simulink model "sampleModel2088"  (R2023a)
settings: Solver=VariableStepAuto  StartTime=0.0  StopTime=10.0  RelTol=1e-3
libraries: simulink x4, hdlsllib x4
settings Model: Creator=user1  LastModifiedBy=user1

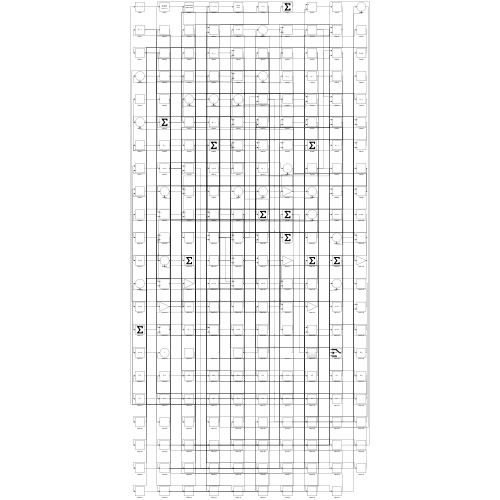
[thumbnail: Simulink's stored preview of the top-level diagram]
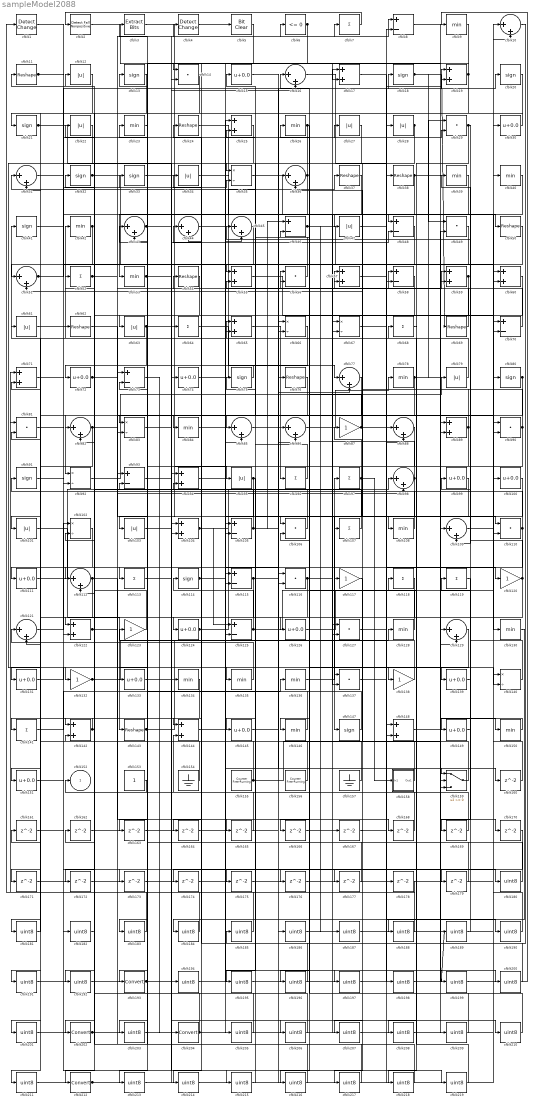
== system sampleModel2088 ==
  cfblk1 : simulink/Logic and Bit Operations/Detect Change  vinit=0  OutDataTypeStr=boolean
      settings: LibrarySourceBlock=|
      | hdlsllib/Logic and Bit
      | Operations/Detect
      | Change
  cfblk{10,16,31,36,43..45,51,77,82,85..86,88,98,109,112,121,129} (18 alike) : Sum  Inputs=|++
  cfblk{15,30,72,74,99..100,111,124,126,131,133,139,145,149,151} (15 alike) : Bias  Bias=0.0  SaturateOnIntegerOverflow=off
  cfblk{12,22,27..28,34,47,61,63,79,95,101,103} (12 alike) : Abs  SaturateOnIntegerOverflow=off
  cfblk{35,66..67,83,92,102,140} (7 alike) : Product  Inputs=*/  RndMeth=Zero  SaturateOnIntegerOverflow=on
  cfblk{17,19,25,55,57,59..60,65,71,89,94,104,122,142,144,148} (16 alike) : Sum
  cfblk{8,46,48,58,70,73,93,105,115,125} (10 alike) : Sum  Inputs=+-
  cfblk{14,29,49,56,81,90,106,110,116,127,137} (11 alike) : DotProduct  OutDataTypeStr=Inherit: Inherit via internal rule
  cfblk{7,52,64,68,96..97,107,113,118..119,141} (11 alike) : Sum  Inputs=+
  cfblk{9,23,26,39..40,42,53,78,84,108,128,130,134..136,146,150} (17 alike) : MinMax
  cfblk{11,24,37..38,50,54,62,69,76,143} (10 alike) : Reshape
  cfblk{13,18,20..21,32..33,41,75,80,91,114,147} (12 alike) : Signum
  cfblk{87,117,120,123,132,138} (6 alike) : Gain
  cfblk153 : Constant  SampleTime=-1
  cfblk154 : Ground
  cfblk155 : hdlsllib/Sources/Counter Free-Running  NumBits=16  tsamp=-1
  cfblk156 : hdlsllib/Sources/Counter Free-Running  NumBits=16  tsamp=-1
  cfblk157 : Ground
  cfblk158 : Subsystem
      settings: LibrarySourceBlock=|
      | hdlsllib/Ports &
      | Subsystems/Subsystem
  cfblk159 : Switch  SaturateOnIntegerOverflow=off  InputSameDT=off
  cfblk{160..179} (20 alike) : Delay  SampleTime=1
  cfblk{180..192,194..201,203,205..211,213..219} (36 alike) : DataTypeConversion  OutDataTypeStr=uint8  SaturateOnIntegerOverflow=off  RndMeth=Floor
  cfblk{193,202,204,212} (4 alike) : DataTypeConversion  SaturateOnIntegerOverflow=off  RndMeth=Floor
  cfblk2 : hdlsllib/Logic and Bit Operations/Detect Fall Nonpositive  vinit=0  OutDataTypeStr=boolean
  cfblk3 : simulink/Logic and Bit Operations/Extract Bits  bitsToExtract=Upper half  numBits=8  bitIdxRange=[0 7]  outScalingMode=Preserve fixed-point scaling
      settings: LibrarySourceBlock=|
      | hdlsllib/Logic and Bit
      | Operations/Extract Bits
  cfblk4 : simulink/Logic and Bit Operations/Detect Change  vinit=0  OutDataTypeStr=boolean
      settings: LibrarySourceBlock=|
      | hdlsllib/Logic and Bit
      | Operations/Detect
      | Change
  cfblk5 : simulink/Logic and Bit Operations/Bit Clear  iBit=0
      settings: LibrarySourceBlock=|
      | hdlsllib/Logic and Bit
      | Operations/Bit Clear
  cfblk6 : hdlsllib/Logic and Bit Operations/Compare To Zero  relop=<=  OutDataTypeStr=boolean
  cfblk152 : Outport  VectorParamsAs1DForOutWhenUnconnected=off
  wires:
  cfblk64/1 -> cfblk77/1
  cfblk99/1 -> cfblk147/1
  cfblk54/1 -> cfblk95/1
  cfblk74/1 -> cfblk37/1
  cfblk80/1 -> cfblk92/1, cfblk83/1
  cfblk136/1 -> cfblk97/1
  cfblk79/1 -> cfblk41/1
  cfblk22/1 -> cfblk132/1
  cfblk65/1 -> cfblk96/1
  cfblk35/1 -> cfblk50/1
  cfblk37/1 -> cfblk53/1
  cfblk7/1 -> cfblk2/1
  cfblk75/1 -> cfblk72/1
  cfblk12/1 -> cfblk101/1
  cfblk63/1 -> cfblk106/1, cfblk83/2
  cfblk3/1 -> cfblk137/1
  cfblk32/1 -> cfblk55/1, cfblk192/1
  cfblk135/1 -> cfblk121/1
  cfblk140/1 -> cfblk45/1
  cfblk89/1 -> cfblk103/1, cfblk56/2, cfblk213/1
  cfblk158/1(Out1) -> cfblk26/1
  cfblk134/1 -> cfblk202/1
  cfblk131/1 -> cfblk139/1
  cfblk19/1 -> cfblk111/1, cfblk14/1
  cfblk73/1 -> cfblk204/1
  cfblk114/1 -> cfblk45/2, cfblk85/2
  cfblk23/1 -> cfblk113/1
  cfblk72/1 -> cfblk18/1, cfblk59/1, cfblk98/2
  cfblk56/1 -> cfblk31/1
  cfblk27/1 -> cfblk85/1
  cfblk86/1 -> cfblk78/1
  cfblk55/1 -> cfblk130/1
  cfblk70/1 -> cfblk56/1
  cfblk38/1 -> cfblk63/1, cfblk170/1
  cfblk109/1 -> cfblk70/1
  cfblk116/1 -> cfblk98/1, cfblk181/1
  cfblk143/1 -> cfblk128/1, cfblk16/2
  cfblk122/1 -> cfblk142/1, cfblk54/1
  cfblk43/1 -> cfblk6/1, cfblk8/1
  cfblk120/1 -> cfblk57/2, cfblk203/1
  cfblk110/1 -> cfblk91/1, cfblk201/1
  cfblk111/1 -> cfblk86/1
  cfblk150/1 -> cfblk149/1
  cfblk1/1 -> cfblk60/2
  cfblk87/1 -> cfblk28/1, cfblk46/2
  cfblk128/1 -> cfblk16/1
  cfblk157/1 -> cfblk142/2
  cfblk30/1 -> cfblk21/1
  cfblk85/1 -> cfblk159/1
  cfblk104/1 -> cfblk108/1, cfblk159/3, cfblk125/1, cfblk110/2
  cfblk61/1 -> cfblk42/1
  cfblk41/1 -> cfblk33/1
  cfblk48/1 -> cfblk122/1
  cfblk50/1 -> cfblk122/2
  cfblk69/1 -> cfblk58/1
  cfblk139/1 -> cfblk99/1
  cfblk71/1 -> cfblk140/2
  cfblk101/1 -> cfblk143/1
  cfblk141/1 -> cfblk136/1
  cfblk34/1 -> cfblk137/2
  cfblk159/1 -> cfblk57/1
  cfblk125/1 -> cfblk117/1, cfblk34/1
  cfblk155/1 -> cfblk109/1, cfblk22/1
  cfblk142/1 -> cfblk141/1, cfblk102/2
  cfblk138/1 -> cfblk123/1
  cfblk16/1 -> cfblk88/1
  cfblk133/1 -> cfblk74/1
  cfblk21/1 -> cfblk94/1, cfblk47/1
  cfblk124/1 -> cfblk17/1, cfblk200/1
  cfblk18/1 -> cfblk69/1, cfblk49/1
  cfblk52/1 -> cfblk4/1, cfblk35/2
  cfblk132/1 -> cfblk76/1, cfblk7/1
  cfblk105/1 -> cfblk62/1, cfblk20/1, cfblk46/1
  cfblk77/1 -> cfblk146/1
  cfblk42/1 -> cfblk92/2, cfblk51/1
  cfblk90/1 -> cfblk36/2, cfblk51/2, cfblk125/2
  cfblk66/1 -> cfblk212/1
  cfblk24/1 -> cfblk70/2
  cfblk115/1 -> cfblk77/2, cfblk59/2, cfblk191/1
  cfblk44/1 -> cfblk116/2
  cfblk82/1 -> cfblk151/1, cfblk110/1
  cfblk57/1 -> cfblk19/1
  cfblk107/1 -> cfblk24/1
  cfblk112/1 -> cfblk168/1, cfblk211/1
  cfblk153/1 -> cfblk152/1
  cfblk26/1 -> cfblk126/1, cfblk31/2, cfblk174/1
  cfblk108/1 -> cfblk52/1
  cfblk95/1 -> cfblk115/2, cfblk175/1
  cfblk156/1 -> cfblk13/1
  cfblk5/1 -> cfblk43/2
  cfblk100/1 -> cfblk145/1
  cfblk92/1 -> cfblk79/1
  cfblk59/1 -> cfblk124/1, cfblk82/1
  cfblk154/1 -> cfblk61/1
  cfblk4/1 -> cfblk5/1
  cfblk78/1 -> cfblk112/1, cfblk150/1, cfblk29/1
  cfblk62/1 -> cfblk90/2
  cfblk2/1 -> cfblk159/2
  cfblk20/1 -> cfblk131/1
  cfblk13/1 -> cfblk112/2
  cfblk97/1 -> cfblk158/1(In1), cfblk87/1, cfblk166/1
  cfblk8/1 -> cfblk89/1
  cfblk98/1 -> cfblk55/2, cfblk195/1
  cfblk46/1 -> cfblk100/1, cfblk187/1
  cfblk126/1 -> cfblk30/1
  cfblk29/1 -> cfblk109/2, cfblk208/1
  cfblk17/1 -> cfblk120/1
  cfblk121/1 -> cfblk102/1
  cfblk83/1 -> cfblk64/1
  cfblk106/1 -> cfblk12/1
  cfblk31/1 -> cfblk135/1
  cfblk146/1 -> cfblk65/1
  cfblk123/1 -> cfblk11/1
  cfblk51/1 -> cfblk19/2, cfblk29/2
  cfblk58/1 -> cfblk133/1
  cfblk36/1 -> cfblk104/2, cfblk35/1
  cfblk6/1 -> cfblk65/2, cfblk44/2
  cfblk11/1 -> cfblk48/1, cfblk176/1
  cfblk33/1 -> cfblk105/2
  cfblk25/1 -> cfblk193/1
  cfblk9/1 -> cfblk17/2
  cfblk76/1 -> cfblk121/2
  cfblk94/1 -> cfblk115/1
  cfblk145/1 -> cfblk27/1
  cfblk28/1 -> cfblk107/1, cfblk84/1
  cfblk60/1 -> cfblk144/1
  cfblk96/1 -> cfblk15/1
  cfblk103/1 -> cfblk138/1
  cfblk147/1 -> cfblk3/1
  cfblk53/1 -> cfblk48/2, cfblk165/1
  cfblk149/1 -> cfblk119/1
  cfblk15/1 -> cfblk160/1
  cfblk160/1 -> cfblk60/1
  cfblk162/1 -> cfblk116/1
  cfblk88/1 -> cfblk163/1
  cfblk49/1 -> cfblk164/1
  cfblk164/1 -> cfblk36/1
  cfblk165/1 -> cfblk144/2
  cfblk166/1 -> cfblk58/2
  cfblk168/1 -> cfblk94/2
  cfblk119/1 -> cfblk169/1
  cfblk169/1 -> cfblk43/1
  cfblk102/1 -> cfblk171/1
  cfblk171/1 -> cfblk86/2
  cfblk14/1 -> cfblk172/1
  cfblk172/1 -> cfblk105/1
  cfblk91/1 -> cfblk173/1
  cfblk174/1 -> cfblk8/2
  cfblk175/1 -> cfblk90/1
  cfblk176/1 -> cfblk89/2
  cfblk117/1 -> cfblk177/1
  cfblk177/1 -> cfblk104/1
  cfblk137/1 -> cfblk178/1
  cfblk178/1 -> cfblk1/1
  cfblk113/1 -> cfblk179/1
  cfblk179/1 -> cfblk23/1
  cfblk161/1 -> cfblk180/1
  cfblk180/1 -> cfblk44/1
  cfblk181/1 -> cfblk161/1
  cfblk81/1 -> cfblk182/1
  cfblk182/1 -> cfblk162/1
  cfblk45/1 -> cfblk183/1
  cfblk183/1 -> cfblk81/1
  cfblk130/1 -> cfblk184/1
  cfblk184/1 -> cfblk81/2
  cfblk10/1 -> cfblk185/1
  cfblk185/1 -> cfblk71/2
  cfblk186/1 -> cfblk10/1
  cfblk187/1 -> cfblk10/2
  cfblk39/1 -> cfblk188/1
  cfblk188/1 -> cfblk71/1
  cfblk189/1 -> cfblk39/1
  cfblk67/1 -> cfblk190/1
  cfblk190/1 -> cfblk140/1
  cfblk191/1 -> cfblk67/1
  cfblk192/1 -> cfblk67/2
  cfblk193/1 -> cfblk189/1, cfblk49/2, cfblk210/1
  cfblk163/1 -> cfblk194/1
  cfblk194/1 -> cfblk25/1
  cfblk195/1 -> cfblk25/2
  cfblk129/1 -> cfblk196/1
  cfblk196/1 -> cfblk114/1
  cfblk84/1 -> cfblk197/1
  cfblk197/1 -> cfblk129/1
  cfblk47/1 -> cfblk198/1
  cfblk198/1 -> cfblk129/2
  cfblk127/1 -> cfblk199/1
  cfblk199/1 -> cfblk9/1
  cfblk200/1 -> cfblk127/1
  cfblk201/1 -> cfblk127/2
  cfblk202/1 -> cfblk186/1, cfblk167/1, cfblk88/2
  cfblk203/1 -> cfblk134/1
  cfblk204/1 -> cfblk82/2, cfblk80/1
  cfblk144/1 -> cfblk205/1
  cfblk205/1 -> cfblk73/1
  cfblk173/1 -> cfblk206/1
  cfblk206/1 -> cfblk73/2
  cfblk118/1 -> cfblk207/1
  cfblk207/1 -> cfblk38/1
  cfblk208/1 -> cfblk118/1
  cfblk148/1 -> cfblk209/1
  cfblk209/1 -> cfblk106/2
  cfblk210/1 -> cfblk148/1
  cfblk211/1 -> cfblk148/2
  cfblk212/1 -> cfblk14/2, cfblk40/1
  cfblk213/1 -> cfblk66/1
  cfblk170/1 -> cfblk214/1
  cfblk214/1 -> cfblk66/2
  cfblk93/1 -> cfblk215/1
  cfblk215/1 -> cfblk75/1
  cfblk40/1 -> cfblk216/1
  cfblk216/1 -> cfblk93/1
  cfblk167/1 -> cfblk217/1
  cfblk217/1 -> cfblk93/2
  cfblk68/1 -> cfblk218/1
  cfblk218/1 -> cfblk32/1
  cfblk151/1 -> cfblk219/1
  cfblk219/1 -> cfblk68/1

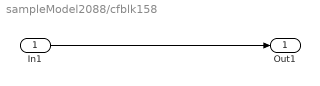
== system sampleModel2088/cfblk158 ==
  In1 : Inport
  Out1 : Outport
  wires:
  In1/1 -> Out1/1
